simulink model "LQRp_c"  (R2015b)
settings: Solver=VariableStepAuto  StartTime=0.0  StopTime=10.0  RelTol=1e-3
undefined symbols (not defined in the file): LQR_K, LQR_N
settings Model: Creator=mgreiff  LastModifiedBy=mgreiff

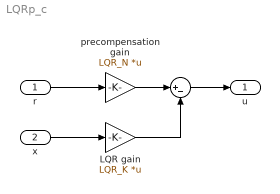
== system LQRp_c ==
  r : Inport  PortDimensions=1
  x : Inport  Port=2  PortDimensions=3
  " " : Sum  Inputs=|+-
  LQR gain : Gain  Gain=LQR_K  Multiplication=Matrix(K*u)
  precompensation gain : Gain  Gain=LQR_N  Multiplication=Matrix(K*u)
  u : Outport  PortDimensions=1
  wires:
  " "/1 -> u/1
  r/1 -> precompensation gain/1
  LQR gain/1 -> " "/2
  precompensation gain/1 -> " "/1
  x/1 -> LQR gain/1
